simulink model "Sim_Multi"  (R2016b)
settings: Solver=ode3  StartTime=0.0  StopTime=sim_time  FixedStep=t_sim  MaxStep=t_control  RelTol=1e-5  EnableMultiTasking=on
values from neighbouring files (symbols this model uses):
  Att_init = [0;0;0] * d2r    [Init_Multi.m]
  Blade_flapping = 0    [Init_Multi.m]
  C_D = 0.40    (= 0.4)    [Init_Multi.m]
  CoG_nominal = [0;0;0.001]    [Init_Multi.m]
  CoG_real = [0;0;0.001]    [Init_Multi.m]
  Coriolis_correction = 1    [Init_Multi.m]
  d2r = pi/180    (= 0.0174532925199)    [Init_Multi.m]
  Dyn_thrust = 0    [Init_Multi.m]
  g = 9.80665    [Init_Multi.m]
  J_nominal = [Jxx Jxy Jxz;Jyx Jyy Jyz;Jzx Jzy Jzz]    [Init_Multi.m]
  J_real = [Jxx Jxy Jxz;Jyx Jyy Jyz;Jzx Jzy Jzz]    [Init_Multi.m]
  k1 = -1.125    [Init_Multi.m]
  k2 = -1.372    [Init_Multi.m]
  k3 = -1.718    [Init_Multi.m]
  k4 = -0.655    [Init_Multi.m]
  k_a1s = 1.5 / 4.0    (= 0.375)    [Init_Multi.m]
  k_beta = 0.23    [Init_Multi.m]
  kappa = 1.00    (= 1)    [Init_Multi.m]
  Kff_1 = 0.7*[1;1;0.95]    [Init_Multi.m]
  Ki_1 = 10*[1;1;1.5]    [Init_Multi.m]
  Kp_1 = 15*[1;1;1.5]    [Init_Multi.m]
  mass_nominal = 0.550    (= 0.55)    [Init_Multi.m]
  mass_real = 0.550    (= 0.55)    [Init_Multi.m]
  max_thrust = max_thrust + (MotorMatrix_nominal(i,7)*MotorMatrix_nominal(i,12)+MotorMatrix_nominal(i,8)*MotorMatrix_nominal(i,12)^2)    [Init_Multi.m]
  MaxRate_cmd = [360;360;120] * d2r    [Init_Multi.m]
  min_thrust = min_thrust + (MotorMatrix_nominal(i,7)*MotorMatrix_nominal(i,11)+MotorMatrix_nominal(i,8)*MotorMatrix_nominal(i,11)^2)    [Init_Multi.m]
  MotorMap = B' * inv(B * B')    [Init_Multi.m]
  MotorMatrix_nominal = [045 , 0.170 , -0.028 , -1 , 1.0 , 0.010 , [9.6820 , 0.010872]*1e-5 , [1.4504 , 0.0016312]*1e-6 , 0000 , 6000 , [0.0 , 0.0 , 0.0] , 8*2.54/100 , 11/1000;                         135 , 0.170 , -0.028 , +1 , 1.0 , 0.010 , [9.6820 , 0.010872]*1e-5 , [1.4504 , 0.0016312]*1e-6 , 0000 , 6000 , [0.0 , 0.0 , 0.0] , 8*2.54/100 , 11/1000;                         225 , 0.170 , -0.028 , -1 , 1.0 , 0.010 , [9. ...(+284 chars)    [Init_Multi.m]
  MotorMatrix_real = [045 , 0.170 , -0.028 , -1 , 1.0 , 0.010 , [9.6820 , 0.010872]*1e-5 , [1.4504 , 0.0016312]*1e-6 , 0000 , 6000 , [0.0 , 0.0 , 0.0] , 8*2.54/100 , 11/1000;                      135 , 0.170 , -0.028 , +1 , 1.0 , 0.010 , [9.6820 , 0.010872]*1e-5 , [1.4504 , 0.0016312]*1e-6 , 0000 , 6000 , [0.0 , 0.0 , 0.0] , 8*2.54/100 , 11/1000;                      225 , 0.170 , -0.028 , -1 , 1.0 , 0.010 , [9.6820 , ...(+275 chars)    [Init_Multi.m]
  Noise_flag = 0    [Init_Multi.m]
  omega_init = [0;0;0]    [Init_Multi.m]
  q_init = rpy2quat(Att_init)    [Init_Multi.m]
  r2d = 180/pi    (= 57.2957795131)    [Init_Multi.m]
  rho = 1.225    [Init_Multi.m]
  rpm2radpersec = 2*pi/60    (= 0.10471975512)    [Init_Multi.m]
  rpm_init = 3104.5025852    [Init_Multi.m]
  Surface_params = [a;b;c]    [Init_Multi.m]
  t_control = 1/500    (= 0.002)    [Init_Multi.m]
  t_sim = t_control/2    (= 0.001)    [Init_Multi.m]
  thrust_gain = (max_thrust - min_thrust) / 1000    (= 0)    [Init_Multi.m]
  thrust_offset = min_thrust    (= 0)    [Init_Multi.m]
  thrust_reserve = 0.10    (= 0.1)    [Init_Multi.m]
  v_h = 4.0    (= 4)    [Init_Multi.m]
  Vb_init = [0;0;0]    [Init_Multi.m]
  Vi_init = R_IB_init' * Vb_init    [Init_Multi.m]
  Xi_init = [0;0;0]    [Init_Multi.m]
undefined symbols (not defined in the file or in its folder): DiscIntNeverNeededParam, rpy2quat, thrust2rpm
libraries: simulink x17
(part 1 of 4)
settings Model: Creator=JV  LastModifiedBy=vervoorst
settings DataIOCC: LimitDataPoints=on  SaveFormat=Array  SignalLoggingSaveFormat=ModelDataLogs
settings OptimizationCC: ExpressionDepthLimit=2147483647  InitFltsAndDblsToZero=on  LifeSpan=inf
settings DebuggingCC: UnderspecifiedInitializationDetection=Classic  MergeDetectMultiDrivingBlocksExec=none  SolverPrmCheckMsg=warning  FcnCallInpInsideContextMsg=warning  StateNameClashWarn=warning  SFUnexpectedBacktrackingDiag=warning  SFNoUnconditionalDefaultTransitionDiag=warning  SFExecutionAtInitializationDiag=none
settings HardwareCC: ProdBitPerPointer=32  ProdBitPerSizeT=32  ProdBitPerPtrDiffT=32  ProdLargestAtomicFloat=None  ProdIntDivRoundTo=Undefined  ProdEndianess=Unspecified  ProdWordSize=32  ProdHWDeviceType=32-bit Generic
settings ModelReferenceCC: PropagateSignalLabelsOutOfModel=off
settings GRTTargetCC: TargetLangStandard=C89/C90 (ANSI)  GeneratePreprocessorConditionals=Disable all  CombineOutputUpdateFcns=off  GRTInterface=on
settings ConfigComp: CovMetricSettings=dw  CovHtmlReporting=on  CovSaveCumulativeToWorkspaceVar=on  CovSaveSingleToWorkspaceVar=on  CovExternalEMLEnable=off  CovSFcnEnable=off

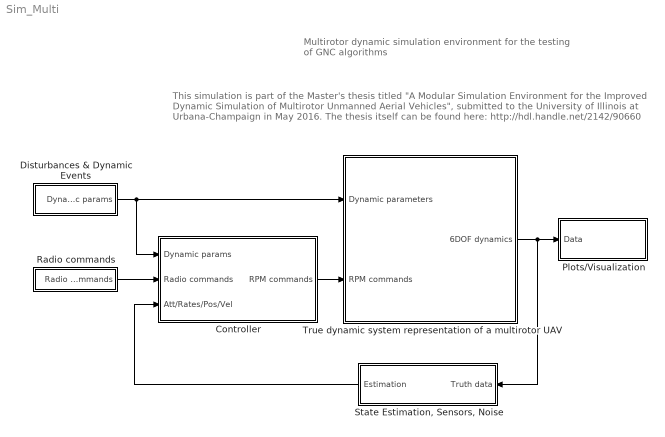
== system Sim_Multi ==
  note: This simulation is part of the Master's thesis titled "A Modular Simulation Environment for the Improved Dynamic Simulation
      | of Multirotor Unmanned Aerial Vehicles", submitted to the University of Illinois at Urbana-Champaign in May 2016.
      | The thesis itself can be found here: http://hdl.handle.net/2142/90660
  note: Multirotor dynamic simulation environment
      | for the testing of GNC algorithms
  Controller : Subsystem
  Disturbances & Dynamic Events : Subsystem
  Plots/Visualization : Subsystem
  Radio commands : Subsystem
  "State Estimation, Sensors, Noise" : Subsystem
  True dynamic system representation of a multirotor UAV : Subsystem
  wires:
  True dynamic system representation of a multirotor UAV/1(6DOF dynamics) -> Plots/Visualization/1(Data), "State Estimation, Sensors, Noise"/1(Truth data)
  Radio commands/1(Radio commands) -> Controller/2(Radio commands)
  "State Estimation, Sensors, Noise"/1(Estimation) -> Controller/3(Att/Rates/Pos/Vel)
  Controller/1(RPM commands) -> True dynamic system representation of a multirotor UAV/2(RPM commands)
  Disturbances & Dynamic Events/1(Dynamic params) -> True dynamic system representation of a multirotor UAV/1(Dynamic parameters), Controller/1(Dynamic params)

== system Sim_Multi/Controller ==
  note: All system parameters used in this block are the nominal parameters
      | that the controller is given about the system.
      | The true parameters of the dynamic system such as mass, inertia,
      | motor mapping matrix, ... may differ from these values.
  Dynamic params : Inport
  Radio commands : Inport  Port=2
  Att/Rates/Pos/Vel : Inport  Port=3
  Controller Structure : Subsystem
  Mapping thrust to rpm and saturation : Subsystem
  Motor mapping : Subsystem
  Reshape : Reshape  OutputDimensionality=Column vector (2-D)
  RPM commands : Outport
  tag scope: RPM_commands=global
  wires:
  Att/Rates/Pos/Vel/1 -> Controller Structure/2(Att/Rates/Pos/Vel)
  Controller Structure/1(Torques/thrust cmd) -> Motor mapping/1(Torques/thrust cmd)
  Radio commands/1 -> Controller Structure/1(Radio commands)
  Reshape/1 -> RPM commands/1
  Dynamic params/1 -> Controller Structure/3(Dynamic params), Mapping thrust to rpm and saturation/2(Dynamic parameters)
  Mapping thrust to rpm and saturation/1(RPM_cmd) -> [RPM_commands], Reshape/1
  Motor mapping/1(Thrust cmds) -> Mapping thrust to rpm and saturation/1(Thrust_cmds)

== system Sim_Multi/Disturbances & Dynamic Events ==
  Bus Creator : BusCreator  Inputs=12
  Constant : Constant  Value=MotorMatrix_real
  Constant1 : Constant  Value=CoG_real
  Constant2 : Constant  Value=mass_real
  Constant3 : Constant  Value=J_real
  Constant4 : Constant  Value=MotorMatrix_nominal
  Constant5 : Constant  Value=CoG_nominal
  Constant6 : Constant  Value=mass_nominal
  Constant7 : Constant  Value=J_nominal
  Disturbance (forces) : Constant  Value=0*[1;1;1]
  Disturbance (torques) : Constant  Value=0*[1;1;1]
  Surface area params : Constant  Value=Surface_params
  Wind vector : Constant  Value=[0;0;0]
  Dynamic params : Outport
  wires:
  Bus Creator/1 -> Dynamic params/1
  Constant/1 -> Bus Creator/1  "MotorMatrix_real"
  Constant1/1 -> Bus Creator/2  "CoG_real"
  Constant2/1 -> Bus Creator/3  "mass_real"
  Constant3/1 -> Bus Creator/4  "J_real"
  Surface area params/1 -> Bus Creator/12  "Surface_params"
  Disturbance (torques)/1 -> Bus Creator/11  "Moment_disturb"
  Disturbance (forces)/1 -> Bus Creator/10  "Force_disturb"
  Wind vector/1 -> Bus Creator/9  "Wind_i"
  Constant4/1 -> Bus Creator/5  "MotorMatrix_nominal"
  Constant5/1 -> Bus Creator/6  "CoG_nominal"
  Constant6/1 -> Bus Creator/7  "mass_nominal"
  Constant7/1 -> Bus Creator/8  "J_nominal"

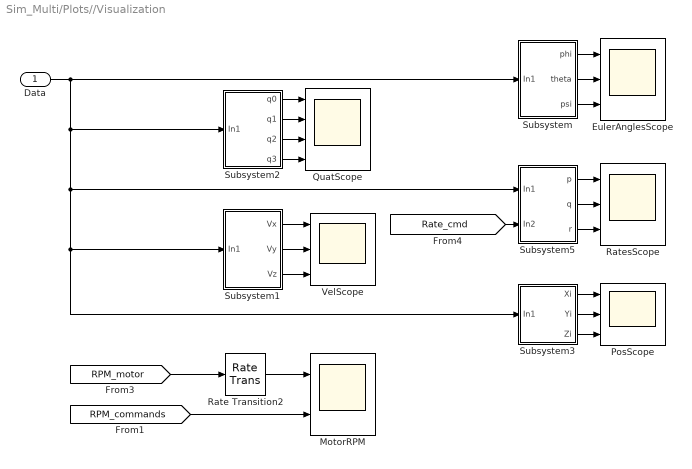
== system Sim_Multi/Plots//Visualization ==
  Data : Inport
  EulerAnglesScope : Scope  NumInputPorts=3
  MotorRPM : Scope  NumInputPorts=2
  PosScope : Scope  NumInputPorts=3
  QuatScope : Scope  NumInputPorts=4
  Rate Transition2 : RateTransition
  RatesScope : Scope  NumInputPorts=3
  Subsystem : Subsystem
  Subsystem1 : Subsystem
  Subsystem2 : Subsystem
  Subsystem3 : Subsystem
  Subsystem5 : Subsystem
  VelScope : Scope  NumInputPorts=3
  wires:
  Data/1 -> Subsystem3/1(In1), Subsystem1/1(In1), Subsystem5/1(In1), Subsystem2/1(In1), Subsystem/1(In1)
  Subsystem/1(phi) -> EulerAnglesScope/1
  Subsystem/2(theta) -> EulerAnglesScope/2
  Subsystem/3(psi) -> EulerAnglesScope/3
  Subsystem2/1(q0) -> QuatScope/1
  Subsystem2/2(q1) -> QuatScope/2
  Subsystem2/3(q2) -> QuatScope/3
  Subsystem2/4(q3) -> QuatScope/4
  Subsystem1/1(Vx) -> VelScope/1
  Subsystem1/2(Vy) -> VelScope/2
  Subsystem1/3(Vz) -> VelScope/3
  Subsystem3/2(Yi) -> PosScope/2
  Subsystem3/3(Zi) -> PosScope/3
  Subsystem3/1(Xi) -> PosScope/1
  Subsystem5/1(p) -> RatesScope/1
  Subsystem5/2(q) -> RatesScope/2
  Subsystem5/3(r) -> RatesScope/3
  [Rate_cmd] -> Subsystem5/2(In2)
  [RPM_commands] -> MotorRPM/2
  [RPM_motor] -> Rate Transition2/1
  Rate Transition2/1 -> MotorRPM/1

== system Sim_Multi/Radio commands ==
  Rate Transition : RateTransition  OutPortSampleTime=t_control
  Rate commands : Subsystem
  Radio commands : Outport
  wires:
  Rate commands/1(Rate commands) -> Rate Transition/1
  Rate Transition/1 -> Radio commands/1

== system Sim_Multi/State Estimation, Sensors, Noise ==
  Truth data : Inport
  Rate Transition : RateTransition  OutPortSampleTime=t_control
  Sensor models : Subsystem
  State estimation : Subsystem
  Estimation : Outport
  wires:
  State estimation/1(Att/Pos/Vel/Accel) -> Rate Transition/1
  Sensor models/1(Corrupted) -> State estimation/1(Sensors)
  Truth data/1 -> Sensor models/1(Truth)
  Rate Transition/1 -> Estimation/1

== system Sim_Multi/True dynamic system representation of a multirotor UAV ==
  Dynamic parameters : Inport
  RPM commands : Inport  Port=2
  6DOF model : Subsystem
  Bus Creator : BusCreator  Inputs=10
  Bus Selector : BusSelector  OutputSignals=mass_real,J_real
  Force/Moment computation : Subsystem
  Rate Transition : RateTransition  OutPortSampleTime=t_sim
  Rate Transition1 : RateTransition  X0=rpm_init  OutPortSampleTime=t_sim
  6DOF dynamics : Outport
  wires:
  RPM commands/1 -> Rate Transition1/1
  Bus Creator/1 -> Force/Moment computation/1(6DOF dynamics), 6DOF dynamics/1
  Dynamic parameters/1 -> Rate Transition/1
  6DOF model/1(X_i [m]) -> Bus Creator/1  "X_i"
  6DOF model/2(V_i [m/s]) -> Bus Creator/2  "V_i"
  6DOF model/3(V_b [m/s]) -> Bus Creator/3  "V_b"
  6DOF model/4(a_b [m/s^2]) -> Bus Creator/4  "a_b"
  Bus Selector/2 -> 6DOF model/4(Inertia [kgm^2])  "<J_real>"
  Bus Selector/1 -> 6DOF model/3(Mass [kg])  "<mass_real>"
  Force/Moment computation/1(Total forces) -> 6DOF model/1(Forces [N])
  Force/Moment computation/2(Total moments) -> 6DOF model/2(Moments [Nm])
  Rate Transition1/1 -> Force/Moment computation/2(RPM commands)
  Rate Transition/1 -> Bus Selector/1, Force/Moment computation/3(Dynamic parameters)
  6DOF model/5(a_i [m/s^2]) -> Bus Creator/5  "a_i"
  6DOF model/6(DCM_ib) -> Bus Creator/6  "DCM_ib"
  6DOF model/7(Quaternion q) -> Bus Creator/7  "Quat q"
  6DOF model/8(Euler [rad]) -> Bus Creator/8  "Euler"
  6DOF model/9(omega [rad/s]) -> Bus Creator/9  "omega"
  6DOF model/10(omega_dot [rad/s^2]) -> Bus Creator/10  "omega_dot"

== system Sim_Multi/Controller/Controller Structure ==
  Radio commands : Inport
  Att/Rates/Pos/Vel : Inport  Port=2
  Dynamic params : Inport  Port=3
  Bus Selector : BusSelector  OutputSignals=J_nominal
  Inner-loop control only : Subsystem
  Torques/thrust cmd : Outport
  tag scope: J_control=global
  wires:
  Dynamic params/1 -> Bus Selector/1
  Bus Selector/1 -> [J_control]  "<J_nominal>"
  Radio commands/1 -> Inner-loop control only/2(Radio commands)
  Att/Rates/Pos/Vel/1 -> Inner-loop control only/1(Att/Rates/Pos/Vel)
  Inner-loop control only/1(Control out) -> Torques/thrust cmd/1

== system Sim_Multi/Controller/Mapping thrust to rpm and saturation ==
  Thrust_cmds : Inport
  Dynamic parameters : Inport  Port=2
  Bus Selector1 : BusSelector  OutputSignals=MotorMatrix_nominal
  For Each Subsystem : Subsystem  TreatAsAtomicUnit=on
  Rate Transition : RateTransition  OutPortSampleTime=t_control
  RPM_cmd : Outport
  wires:
  For Each Subsystem/1(RPM_cmd_sat) -> Rate Transition/1
  Dynamic parameters/1 -> Bus Selector1/1
  Bus Selector1/1 -> For Each Subsystem/2(MotorMatrix_nominal)  "<MotorMatrix_nominal>"
  Rate Transition/1 -> RPM_cmd/1
  Thrust_cmds/1 -> For Each Subsystem/1(Thrust_cmds)

== system Sim_Multi/Controller/Motor mapping ==
  note: Overall thrust command is limited to a range
      | of 10...90% of max thrust to still allow room
      | for torque demands needed for maneuvering
  note: The motor mapping matrix used here to transform body axis torque commands
      | into thrust commands for each motor is populated with the nominal arm length
      | and motor position information that the controller thinks are correct, not the
      | actual values used in the true dynamics computation block.
  Torques/thrust cmd : Inport
  Constant1 : Constant  Value=MotorMap
  Demux : Demux  Outputs=[3 1]
  Matrix Multiply1 : Product  Multiplication=Matrix(*)
  Max thrust limit : Subsystem
  Min thrust limit : Subsystem
  Mux : Mux  Inputs=2
  Rate Transition : RateTransition  OutPortSampleTime=t_control
  Saturation Dynamic : simulink/Discontinuities/Saturation Dynamic  OutMin=[]  OutMax=[]  OutDataTypeStr=Inherit: Same as second input  OutDataType=fixdt(1, 16)  OutScaling=2^-10  DoSatur=off
  Thrust cmds : Outport
  wires:
  Constant1/1 -> Matrix Multiply1/1
  Rate Transition/1 -> Thrust cmds/1  "These are thrust demands to each motor"
  Matrix Multiply1/1 -> Rate Transition/1
  Torques/thrust cmd/1 -> Demux/1
  Demux/2 -> Saturation Dynamic/2
  Min thrust limit/1(Out1) -> Saturation Dynamic/3
  Max thrust limit/1(Out1) -> Saturation Dynamic/1
  Saturation Dynamic/1 -> Mux/2
  Demux/1 -> Mux/1
  Mux/1 -> Matrix Multiply1/2

== system Sim_Multi/Plots//Visualization/Subsystem ==
  In1 : Inport
  Bus Selector : BusSelector  OutputSignals=Euler
  Demux : Demux  Outputs=3
  Gain : Gain  Gain=r2d
  phi : Outport
  theta : Outport  Port=2
  psi : Outport  Port=3
  wires:
  Bus Selector/1 -> Gain/1  "<Euler>"
  In1/1 -> Bus Selector/1
  Gain/1 -> Demux/1
  Demux/1 -> phi/1
  Demux/2 -> theta/1
  Demux/3 -> psi/1

== system Sim_Multi/Plots//Visualization/Subsystem1 ==
  In1 : Inport
  Bus Selector : BusSelector  OutputSignals=V_i
  Demux4 : Demux  Outputs=3
  Vx : Outport
  Vy : Outport  Port=2
  Vz : Outport  Port=3
  wires:
  Bus Selector/1 -> Demux4/1  "<V_i>"
  In1/1 -> Bus Selector/1
  Demux4/1 -> Vx/1
  Demux4/2 -> Vy/1
  Demux4/3 -> Vz/1

== system Sim_Multi/Plots//Visualization/Subsystem2 ==
  In1 : Inport
  Bus Selector : BusSelector  OutputSignals=Quat q
  Demux5 : Demux
  q0 : Outport
  q1 : Outport  Port=2
  q2 : Outport  Port=3
  q3 : Outport  Port=4
  wires:
  Bus Selector/1 -> Demux5/1  "<Quat q>"
  In1/1 -> Bus Selector/1
  Demux5/1 -> q0/1
  Demux5/2 -> q1/1
  Demux5/3 -> q2/1
  Demux5/4 -> q3/1

== system Sim_Multi/Plots//Visualization/Subsystem3 ==
  In1 : Inport
  Bus Selector : BusSelector  OutputSignals=X_i
  Demux4 : Demux  Outputs=3
  Xi : Outport
  Yi : Outport  Port=2
  Zi : Outport  Port=3
  wires:
  Bus Selector/1 -> Demux4/1  "<X_i>"
  In1/1 -> Bus Selector/1
  Demux4/1 -> Xi/1
  Demux4/2 -> Yi/1
  Demux4/3 -> Zi/1

== system Sim_Multi/Plots//Visualization/Subsystem5 ==
  In1 : Inport
  In2 : Inport  Port=2
  Bus Selector : BusSelector  OutputSignals=omega
  Demux : Demux  Outputs=3
  Demux1 : Demux  Outputs=3
  Mux : Mux  Inputs=2
  Mux1 : Mux  Inputs=2
  Mux2 : Mux  Inputs=2
  Rate Transition : RateTransition  OutPortSampleTime=t_sim
  p : Outport
  q : Outport  Port=2
  r : Outport  Port=3
  wires:
  Bus Selector/1 -> Demux/1  "<omega>"
  Demux/1 -> Mux1/1
  Demux1/1 -> Mux1/2
  Demux/2 -> Mux/1
  Demux1/2 -> Mux/2
  Demux/3 -> Mux2/1
  Demux1/3 -> Mux2/2
  In1/1 -> Bus Selector/1
  In2/1 -> Rate Transition/1
  Mux1/1 -> p/1
  Mux/1 -> q/1
  Mux2/1 -> r/1
  Rate Transition/1 -> Demux1/1

== system Sim_Multi/Radio commands/Rate commands ==
  note: The signal magnitude for the throttle should be
      | in a range of [0,1000]
  Filter : Subsystem
  Mux : Mux  Inputs=3
  Mux1 : Mux  Inputs=2
  Pitch rate signal : Subsystem
  Rate Transition : RateTransition  OutPortSampleTime=t_control
  Roll rate signal : Subsystem
  Throttle value : Constant  Value=299.9916292904752
  Yaw rate signal : Subsystem
  Rate commands : Outport
  wires:
  Filter/2(theta_dot filtered) -> Mux/2
  Mux1/1 -> Rate commands/1
  Filter/3(psi_dot filtered) -> Mux/3
  Filter/1(phi_dot filtered) -> Mux/1
  Roll rate signal/1(phi) -> Filter/1(Roll rate)
  Mux/1 -> Rate Transition/1
  Pitch rate signal/1(theta) -> Filter/2(Pitch rate)
  Yaw rate signal/1(psi) -> Filter/3(Yaw rate)
  Throttle value/1 -> Mux1/2
  Rate Transition/1 -> Mux1/1

== system Sim_Multi/State Estimation, Sensors, Noise/Sensor models ==
  note: The available sensor outputs are body rates and body accelerations.
      | In the simple case, noise is added to the rate and accel outputs of the 6DOF block to 'simulate' sensor output.
  Truth : Inport
  Acc noise : Subsystem
  Bus Creator : BusCreator  Inputs=9
  Bus Selector : BusSelector  OutputSignals=a_b,omega
  Bus Selector1 : BusSelector  OutputSignals=X_i,V_i,V_b,DCM_ib,Quat q,Euler,omega_dot
  Gain : Gain
  Gain1 : Gain
  Gyro noise : Subsystem
  Noisy acc : Scope
  Noisy omega : Scope
  Sum : Sum
  Sum1 : Sum
  Corrupted : Outport
  wires:
  Truth/1 -> Bus Selector/1, Bus Selector1/1
  Bus Creator/1 -> Corrupted/1
  Sum/1 -> Noisy omega/1, Gain/1  "omega"
  Sum1/1 -> Noisy acc/1, Gain1/1  "a_b"
  Bus Selector1/1 -> Bus Creator/1  "<X_i>"
  Bus Selector1/2 -> Bus Creator/2  "<V_i>"
  Bus Selector1/3 -> Bus Creator/3  "<V_b>"
  Acc noise/1(Noise) -> Sum1/1
  Bus Selector/1 -> Sum1/2  "<a_b>"
  Gain1/1 -> Bus Creator/4  "a_b"
  Bus Selector1/4 -> Bus Creator/5  "<DCM_ib>"
  Bus Selector1/5 -> Bus Creator/6  "<Quat q>"
  Bus Selector1/6 -> Bus Creator/7  "<Euler>"
  Gyro noise/1(Noise) -> Sum/2
  Bus Selector/2 -> Sum/1  "<omega>"
  Gain/1 -> Bus Creator/8  "omega"
  Bus Selector1/7 -> Bus Creator/9  "<omega_dot>"

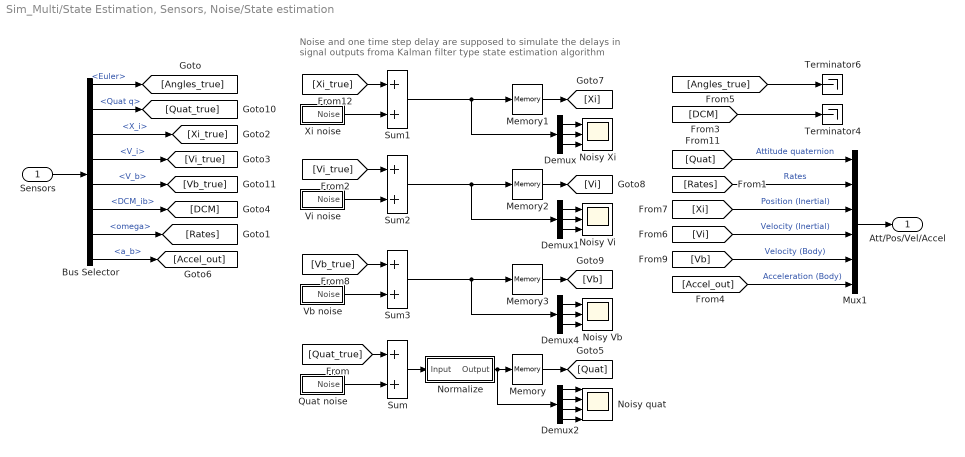
== system Sim_Multi/State Estimation, Sensors, Noise/State estimation ==
  note: Noise and one time step delay are supposed to simulate the delays
      | in signal outputs froma Kalman filter type state estimation algorithm
  Sensors : Inport
  Bus Selector : BusSelector  OutputSignals=Euler,Quat q,X_i,V_i,V_b,DCM_ib,omega,a_b
  Demux : Demux  Outputs=3
  Demux1 : Demux  Outputs=3
  Demux2 : Demux
  Demux4 : Demux  Outputs=3
  Memory : Memory  X0=q_init
  Memory1 : Memory  X0=Xi_init
  Memory2 : Memory  X0=Vi_init
  Memory3 : Memory  X0=Vi_init
  Mux1 : Mux  Inputs=6
  Noisy Vb : Scope  NumInputPorts=3
  Noisy Vi : Scope  NumInputPorts=3
  Noisy Xi : Scope  NumInputPorts=3
  Noisy quat : Scope  NumInputPorts=4
  Normalize : Subsystem
  Quat noise : Subsystem
  Sum{,1..3} (4 alike) : Sum
  Terminator4 : Terminator
  Terminator6 : Terminator
  Vb noise : Subsystem
  Vi noise : Subsystem
  Xi noise : Subsystem
  Att/Pos/Vel/Accel : Outport
  wires:
  Sensors/1 -> Bus Selector/1
  Bus Selector/3 -> [Xi_true]  "<X_i>"
  Bus Selector/4 -> [Vi_true]  "<V_i>"
  Bus Selector/6 -> [DCM]  "<DCM_ib>"
  Bus Selector/7 -> [Rates]  "<omega>"
  Bus Selector/8 -> [Accel_out]  "<a_b>"
  Bus Selector/1 -> [Angles_true]  "<Euler>"
  [Quat] -> Mux1/1  "Attitude quaternion"
  [Rates] -> Mux1/2  "Rates"
  Bus Selector/2 -> [Quat_true]  "<Quat q>"
  [DCM] -> Terminator4/1
  [Angles_true] -> Terminator6/1
  Sum/1 -> Normalize/1(Input)
  Quat noise/1(Noise) -> Sum/2
  [Quat_true] -> Sum/1
  Normalize/1(Output) -> Demux2/1, Memory/1
  Memory/1 -> [Quat]
  Xi noise/1(Noise) -> Sum1/2
  Sum1/1 -> Demux/1, Memory1/1
  Memory1/1 -> [Xi]
  [Xi_true] -> Sum1/1
  Vi noise/1(Noise) -> Sum2/2
  Memory2/1 -> [Vi]
  [Vi_true] -> Sum2/1
  [Xi] -> Mux1/3  "Position (Inertial)"
  [Vi] -> Mux1/4  "Velocity (Inertial)"
  Mux1/1 -> Att/Pos/Vel/Accel/1
  Sum2/1 -> Demux1/1, Memory2/1
  Demux/1 -> Noisy Xi/1
  Demux/2 -> Noisy Xi/2
  Demux/3 -> Noisy Xi/3
  Demux1/1 -> Noisy Vi/1
  Demux1/2 -> Noisy Vi/2
  Demux1/3 -> Noisy Vi/3
  Demux2/1 -> Noisy quat/1
  Demux2/2 -> Noisy quat/2
  Demux2/3 -> Noisy quat/3
  Demux2/4 -> Noisy quat/4
  Vb noise/1(Noise) -> Sum3/2
  Memory3/1 -> [Vb]
  [Vb_true] -> Sum3/1
  Sum3/1 -> Demux4/1, Memory3/1
  Demux4/1 -> Noisy Vb/1
  Demux4/2 -> Noisy Vb/2
  Demux4/3 -> Noisy Vb/3
  Bus Selector/5 -> [Vb_true]  "<V_b>"
  [Vb] -> Mux1/5  "Velocity (Body)"
  [Accel_out] -> Mux1/6  "Acceleration (Body)"

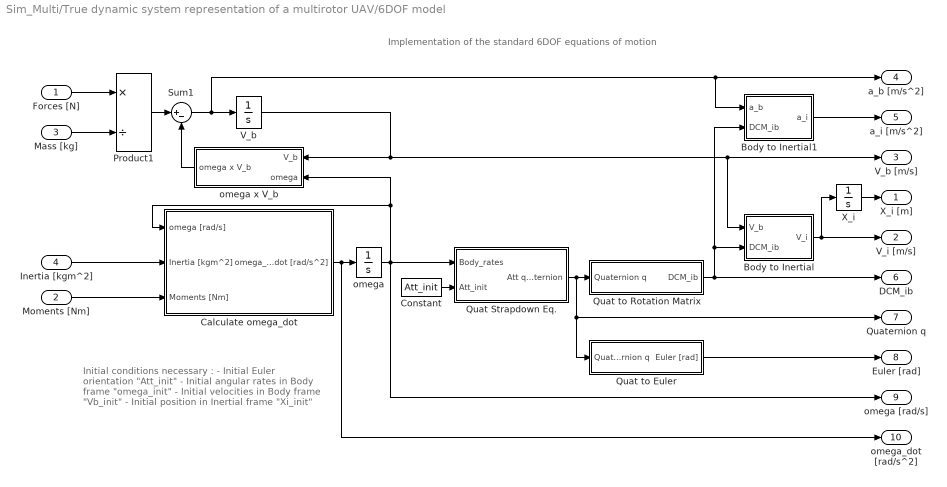
== system Sim_Multi/True dynamic system representation of a multirotor UAV/6DOF model ==
  note: Implementation of the standard 6DOF equations of motion
  note: Initial conditions necessary :
      | - Initial Euler orientation "Att_init"
      | - Initial angular rates in Body frame "omega_init"
      | - Initial velocities in Body frame "Vb_init"
      | - Initial position in Inertial frame "Xi_init"
  Forces [N] : Inport
  Moments [Nm] : Inport  Port=2
  Mass [kg] : Inport  Port=3
  Inertia [kgm^2] : Inport  Port=4
  Body to Inertial : Subsystem
  Body to Inertial1 : Subsystem
  Calculate omega_dot : Subsystem
  Constant : Constant  Value=Att_init
  Product1 : Product  Inputs=*/  SaturateOnIntegerOverflow=on  OutDataTypeStr=Inherit: Same as first input
  Quat Strapdown Eq. : Subsystem
  Quat to Euler : Subsystem
  Quat to Rotation Matrix : Subsystem
  Sum1 : Sum  Inputs=|+-  SaturateOnIntegerOverflow=on
  V_b : Integrator  InitialCondition=Vb_init
  X_i : Integrator  InitialCondition=Xi_init
  omega : Integrator  InitialCondition=omega_init
  omega x V_b : Subsystem
  X_i [m] : Outport
  V_i [m/s] : Outport  Port=2
  V_b [m/s] : Outport  Port=3
  a_b [m/s^2] : Outport  Port=4
  a_i [m/s^2] : Outport  Port=5
  DCM_ib : Outport  Port=6
  Quaternion q : Outport  Port=7
  Euler [rad] : Outport  Port=8
  omega [rad/s] : Outport  Port=9
  omega_dot [rad/s^2] : Outport  Port=10
  wires:
  Forces [N]/1 -> Product1/1
  Mass [kg]/1 -> Product1/2
  Product1/1 -> Sum1/1
  omega x V_b/1(omega x V_b) -> Sum1/2
  V_b/1 -> V_b [m/s]/1, Body to Inertial/1(V_b), omega x V_b/1(V_b)
  Inertia [kgm^2]/1 -> Calculate omega_dot/2(Inertia [kgm^2])
  Moments [Nm]/1 -> Calculate omega_dot/3(Moments [Nm])
  Calculate omega_dot/1(omega_dot [rad/s^2]) -> omega_dot [rad/s^2]/1, omega/1
  omega/1 -> Calculate omega_dot/1(omega [rad/s]), omega x V_b/2(omega), omega [rad/s]/1, Quat Strapdown Eq./1(Body_rates)
  Quat Strapdown Eq./1(Att quaternion) -> Quat to Euler/1(Quaternion q), Quaternion q/1, Quat to Rotation Matrix/1(Quaternion q)
  Quat to Euler/1(Euler [rad]) -> Euler [rad]/1
  Body to Inertial/1(V_i) -> V_i [m/s]/1, X_i/1
  X_i/1 -> X_i [m]/1
  Constant/1 -> Quat Strapdown Eq./2(Att_init)
  Quat to Rotation Matrix/1(DCM_ib) -> Body to Inertial1/2(DCM_ib), Body to Inertial/2(DCM_ib), DCM_ib/1
  Body to Inertial1/1(a_i) -> a_i [m/s^2]/1
  Sum1/1 -> V_b/1, a_b [m/s^2]/1, Body to Inertial1/1(a_b)

== system Sim_Multi/True dynamic system representation of a multirotor UAV/Force//Moment computation ==
  note: Computation of all forces and moments acting on the airframe
  6DOF dynamics : Inport
  RPM commands : Inport  Port=2
  Dynamic parameters : Inport  Port=3
  Bus Selector : BusSelector  OutputSignals=Force_disturb,Moment_disturb
  Compute aerodynamic drag of the airframe in Body axes : Subsystem
  Compute force of gravity in Body axes : Subsystem
  Forces and moments generated by spinning propellers : Subsystem
  Sum{,1..3} (4 alike) : Sum  Inputs=|++
  Total forces : Outport
  Total moments : Outport  Port=2
  wires:
  RPM commands/1 -> Forces and moments generated by spinning propellers/1(RPM_commands)
  6DOF dynamics/1 -> Forces and moments generated by spinning propellers/3(6DOF dynamics), Compute aerodynamic drag of the airframe in Body axes/1(6DOF dynamics), Compute force of gravity in Body axes/1(6DOF dynamics)
  Forces and moments generated by spinning propellers/2(Motor forces) -> Sum/1
  Compute force of gravity in Body axes/1(Gravity force) -> Sum/2
  Dynamic parameters/1 -> Bus Selector/1, Compute aerodynamic drag of the airframe in Body axes/2(Dynamic parameters), Compute force of gravity in Body axes/2(Dynamic parameters), Forces and moments generated by spinning propellers/2(Dynamic parameters)
  Bus Selector/1 -> Sum1/2  "<Force_disturb>"
  Bus Selector/2 -> Sum2/2  "<Moment_disturb>"
  Forces and moments generated by spinning propellers/1(Motor moments) -> Sum2/1
  Sum/1 -> Sum3/1
  Sum3/1 -> Sum1/1
  Compute aerodynamic drag of the airframe in Body axes/1(Drag force) -> Sum3/2
  Sum2/1 -> Total moments/1
  Sum1/1 -> Total forces/1

== system Sim_Multi/Controller/Controller Structure/Inner-loop control only ==
  note: The output of the inner-loop controller is always
      | a set of three commanded torques around the
      | Body axes, roll/pitch/yaw, and an overall thrust
      | command.
      | This is independent of what the structure of the
      | multirotor airframe is assumed to be.
  Att/Rates/Pos/Vel : Inport
  Radio commands : Inport  Port=2
  Conversion stick values to rate commands : Subsystem
  Demux : Demux  Outputs=[4 3 3 3 3 3]
  PI Rate controller : Subsystem
  Terminator{,1..4} (5 alike) : Terminator
  Control out : Outport
  wires:
  Att/Rates/Pos/Vel/1 -> Demux/1
  Demux/3 -> Terminator/1  "Xi"
  Demux/4 -> Terminator1/1  "Vi"
  Demux/5 -> Terminator2/1  "Vb"
  Demux/6 -> Terminator3/1  "a_b"
  Radio commands/1 -> Conversion stick values to rate commands/1(Sticks/Throttle cmd)
  PI Rate controller/1(Control/Throttle out) -> Control out/1
  Demux/2 -> PI Rate controller/2(Rate_est)
  Conversion stick values to rate commands/1(Rates/Throttle cmd) -> PI Rate controller/1(Rates/Throttle cmd)
  Demux/1 -> Terminator4/1

== system Sim_Multi/Controller/Mapping thrust to rpm and saturation/For Each Subsystem ==
  note: The thrust commands from the controller are turned into RPM commands by solving the
      | nominal (quadratic) rpm to thrust equations for RPM.
      | These min and max RPM values are then saturated using the nominal min and max RPM
      | values given for the particular motor/propeller combination.
  Thrust_cmds : Inport  Partition=on  PartitionDimension=1  PartitionWidth=1
  MotorMatrix_nominal : Inport  Port=2  Partition=on  PartitionDimension=1  PartitionWidth=1
  For Each : ForEach  DisableCoverage=on  IndexMode=One-based
  Mux : Mux  Inputs=2
  Saturation Dynamic : simulink/Discontinuities/Saturation Dynamic  OutMin=[]  OutMax=[]  OutDataTypeStr=Inherit: Same as second input  OutDataType=fixdt(1, 16)  OutScaling=2^-10  DoSatur=off
  Saturation limit: no negative thrust : Saturate  UpperLimit=inf  LowerLimit=0
  Selector1 : Selector  InputPortWidth=17  IndexOptions=Index vector (dialog)  Indices=[11]  OutputSizes=1
  Selector2 : Selector  InputPortWidth=17  IndexOptions=Index vector (dialog)  Indices=[12]  OutputSizes=1
  Selector3 : Selector  InputPortWidth=17  IndexOptions=Index vector (dialog)  Indices=[7 8]  OutputSizes=1
  thrust2rpm : MATLABFcn  MATLABFcn=thrust2rpm(u)  OutputDimensions=1
  RPM_cmd_sat : Outport  ConcatenationDimension=1
  wires:
  Selector3/1 -> Mux/1  "Thrust params a1 and a2"
  Thrust_cmds/1 -> Saturation limit: no negative thrust/1
  Mux/1 -> thrust2rpm/1
  thrust2rpm/1 -> Saturation Dynamic/2  "Commanded RPM value for each motor"
  Selector2/1 -> Saturation Dynamic/1  "Nominal max RPM"
  Selector1/1 -> Saturation Dynamic/3  "Nominal min RPM"
  Saturation Dynamic/1 -> RPM_cmd_sat/1
  MotorMatrix_nominal/1 -> Selector1/1, Selector2/1, Selector3/1
  Saturation limit: no negative thrust/1 -> Mux/2

== system Sim_Multi/Controller/Motor mapping/Max thrust limit ==
  Constant : Constant  Value=max_thrust
  Constant2 : Constant  Value=min_thrust
  Gain : Gain  Gain=thrust_reserve
  Sum : Sum  Inputs=|+-
  Sum1 : Sum  Inputs=+-|
  Out1 : Outport
  wires:
  Constant/1 -> Sum1/1, Sum/1
  Sum1/1 -> Out1/1
  Constant2/1 -> Sum/2
  Sum/1 -> Gain/1
  Gain/1 -> Sum1/2

== system Sim_Multi/Controller/Motor mapping/Min thrust limit ==
  Constant : Constant  Value=max_thrust
  Constant2 : Constant  Value=min_thrust
  Gain : Gain  Gain=thrust_reserve
  Sum : Sum  Inputs=|+-
  Sum1 : Sum  Inputs=|++
  Out1 : Outport
  wires:
  Constant/1 -> Sum/1
  Sum1/1 -> Out1/1
  Constant2/1 -> Sum1/2, Sum/2
  Sum/1 -> Gain/1
  Gain/1 -> Sum1/1

== system Sim_Multi/Radio commands/Rate commands/Filter ==
  Roll rate : Inport
  Pitch rate : Inport  Port=2
  Yaw rate : Inport  Port=3
  Transfer Fcn{1..6} (6 alike) : TransferFcn  Denominator=[.01 1]
  phi_dot filtered : Outport
  theta_dot filtered : Outport  Port=2
  psi_dot filtered : Outport  Port=3
  wires:
  Transfer Fcn6/1 -> Transfer Fcn1/1
  Transfer Fcn2/1 -> Transfer Fcn3/1
  Transfer Fcn4/1 -> Transfer Fcn5/1
  Yaw rate/1 -> Transfer Fcn2/1
  Transfer Fcn3/1 -> psi_dot filtered/1
  Pitch rate/1 -> Transfer Fcn4/1
  Transfer Fcn5/1 -> theta_dot filtered/1
  Roll rate/1 -> Transfer Fcn6/1
  Transfer Fcn1/1 -> phi_dot filtered/1

== system Sim_Multi/Radio commands/Rate commands/Pitch rate signal ==
  note: The signal magnitude for the pitch channel should be at most 1.
      | It then gets scaled by a factor of 500 to simulate a PWM output
      | range of [-500,500]
  Add1 : Sum  Inputs=+++
  Add2 : Sum  Inputs=+++
  Constant : Constant  Value=0
  Gain : Gain
  Gain1 : Gain  Gain=0.1
  Gain2 : Gain  Gain=500
  Manual Switch : ManualSwitch  CurrentSetting=0
  Manual Switch1 : ManualSwitch
  Step1 : Step  SampleTime=0
  Step2 : Step  Time=2  After=-2  SampleTime=0
  Step3 : Step  Time=3.5  SampleTime=0
  Step4 : Step  Time=4.5  After=-2  SampleTime=0
  Step5 : Step  Time=5.5  SampleTime=0
  Step6 : Step  Time=3  SampleTime=0
  theta : Outport
  wires:
  Add1/1 -> Gain/1
  Step3/1 -> Add1/1
  Step4/1 -> Add1/2
  Step5/1 -> Add1/3
  Gain2/1 -> theta/1
  Gain/1 -> Manual Switch/1
  Add2/1 -> Gain1/1
  Step1/1 -> Add2/1
  Step2/1 -> Add2/2
  Step6/1 -> Add2/3
  Gain1/1 -> Manual Switch/2
  Manual Switch/1 -> Manual Switch1/1
  Constant/1 -> Manual Switch1/2
  Manual Switch1/1 -> Gain2/1

== system Sim_Multi/Radio commands/Rate commands/Roll rate signal ==
  note: The signal magnitude for the roll channel should be at most 1.
      | It then gets scaled by a factor of 500 to simulate a PWM output
      | range of [-500,500]
  Add : Sum  Inputs=+++
  Constant : Constant  Value=0
  Gain : Gain  Gain=0.1
  Gain2 : Gain  Gain=500
  Manual Switch : ManualSwitch
  Manual Switch1 : ManualSwitch
  Step : Step  Time=0.5  SampleTime=0
  Step1 : Step  Time=1.5  After=-2  SampleTime=0
  Step2 : Step  Time=2.5  SampleTime=0
  Step3 : Step  Time=0.5  SampleTime=0
  phi : Outport
  wires:
  Step/1 -> Add/1
  Step1/1 -> Add/2
  Step2/1 -> Add/3
  Add/1 -> Gain/1
  Gain2/1 -> phi/1
  Gain/1 -> Manual Switch/1
  Manual Switch/1 -> Manual Switch1/1
  Manual Switch1/1 -> Gain2/1
  Constant/1 -> Manual Switch1/2
  Step3/1 -> Manual Switch/2

== system Sim_Multi/Radio commands/Rate commands/Yaw rate signal ==
  note: The signal magnitude for the yaw channel should be at most 1.
      | It then gets scaled by a factor of 500 to simulate a PWM output
      | range of [-500,500]
  Add1 : Sum  Inputs=+++
  Add2 : Sum  Inputs=+++
  Constant : Constant  Value=0
  Gain : Gain  Gain=0.2
  Gain1 : Gain  Gain=0.2
  Gain2 : Gain  Gain=500
  Manual Switch : ManualSwitch  CurrentSetting=0
  Manual Switch1 : ManualSwitch  CurrentSetting=0
  Step1 : Step  Time=2  SampleTime=0
  Step2 : Step  Time=3  After=-2  SampleTime=0
  Step3 : Step  Time=4  SampleTime=0
  Step6 : Step  Time=6.5  SampleTime=0
  Step7 : Step  Time=7.5  After=-2  SampleTime=0
  Step8 : Step  Time=8.5  SampleTime=0
  psi : Outport
  wires:
  Step6/1 -> Add2/1
  Step7/1 -> Add2/2
  Step8/1 -> Add2/3
  Add2/1 -> Gain1/1
  Gain2/1 -> psi/1
  Step1/1 -> Add1/1
  Step2/1 -> Add1/2
  Step3/1 -> Add1/3
  Add1/1 -> Gain/1
  Gain/1 -> Manual Switch/2
  Manual Switch/1 -> Manual Switch1/1
  Manual Switch1/1 -> Gain2/1
  Constant/1 -> Manual Switch1/2
  Gain1/1 -> Manual Switch/1

== system Sim_Multi/State Estimation, Sensors, Noise/Sensor models/Acc noise ==
  Band-Limited White Noise : simulink/Sources/Band-Limited White Noise  Cov=t_sim*57.3*57.3/10000  Ts=t_sim  seed=[25341]
  Constant : Constant  Value=Noise_flag
  Constant1 : Constant  Value=0
  Gain1 : Gain  Gain=0.1
  Gain2 : Gain  Gain=0.08
  Integrator : Integrator
  Sum1 : Sum  Inputs=++|
  Switch : Switch  Criteria=u2 > Threshold
  Uniform Random Number : UniformRandomNumber  Minimum=-.001  Maximum=.001  Seed=657  SampleTime=t_sim
  Noise : Outport
  wires:
  Band-Limited White Noise/1 -> Gain2/1
  Uniform Random Number/1 -> Integrator/1
  Integrator/1 -> Gain1/1
  Switch/1 -> Noise/1
  Constant/1 -> Switch/2
  Constant1/1 -> Switch/3
  Gain2/1 -> Sum1/1
  Gain1/1 -> Sum1/2
  Sum1/1 -> Switch/1

== system Sim_Multi/State Estimation, Sensors, Noise/Sensor models/Gyro noise ==
  Band-Limited White Noise : simulink/Sources/Band-Limited White Noise  Cov=t_sim*57.3*57.3/10000  Ts=t_sim  seed=[23341]
  Constant : Constant  Value=Noise_flag
  Constant1 : Constant  Value=0
  Gain1 : Gain  Gain=0.1
  Gain2 : Gain  Gain=0.07
  Integrator : Integrator
  Sum1 : Sum  Inputs=++|
  Switch : Switch  Criteria=u2 > Threshold
  Uniform Random Number : UniformRandomNumber  Minimum=-.001  Maximum=.001  Seed=338  SampleTime=t_sim
  Noise : Outport
  wires:
  Band-Limited White Noise/1 -> Gain2/1
  Uniform Random Number/1 -> Integrator/1
  Integrator/1 -> Gain1/1
  Switch/1 -> Noise/1
  Constant/1 -> Switch/2
  Constant1/1 -> Switch/3
  Gain2/1 -> Sum1/1
  Gain1/1 -> Sum1/2
  Sum1/1 -> Switch/1

== system Sim_Multi/State Estimation, Sensors, Noise/State estimation/Normalize ==
  Input : Inport
  Divide : Product  Inputs=*/
  norm : Subsystem
  Output : Outport
  wires:
  Input/1 -> Divide/1, norm/1(u)
  norm/1(||u||) -> Divide/2
  Divide/1 -> Output/1

== system Sim_Multi/State Estimation, Sensors, Noise/State estimation/Quat noise ==
  Band-Limited White Noise : simulink/Sources/Band-Limited White Noise  Cov=t_sim*57.3*57.3/10000  Ts=t_sim*30  seed=[23099]
  Constant : Constant  Value=Noise_flag
  Constant1 : Constant  Value=0
  Gain2 : Gain  Gain=0.1
  Rate Transition1 : RateTransition  OutPortSampleTime=t_sim
  Switch : Switch  Criteria=u2 > Threshold
  Noise : Outport
  wires:
  Band-Limited White Noise/1 -> Gain2/1
  Switch/1 -> Noise/1
  Constant/1 -> Switch/2
  Constant1/1 -> Switch/3
  Gain2/1 -> Rate Transition1/1
  Rate Transition1/1 -> Switch/1

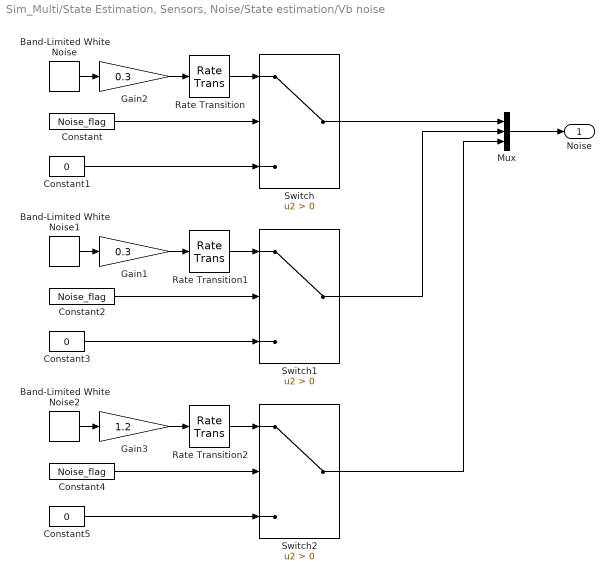
== system Sim_Multi/State Estimation, Sensors, Noise/State estimation/Vb noise ==
  Band-Limited White Noise : simulink/Sources/Band-Limited White Noise  Cov=t_sim*57.3*57.3/10000  Ts=t_sim*10  seed=[21234]
  Band-Limited White Noise1 : simulink/Sources/Band-Limited White Noise  Cov=t_sim*57.3*57.3/10000  Ts=t_sim*10  seed=[21234]
  Band-Limited White Noise2 : simulink/Sources/Band-Limited White Noise  Cov=t_sim*57.3*57.3/10000  Ts=t_sim*10  seed=[21234]
  Constant : Constant  Value=Noise_flag
  Constant1 : Constant  Value=0
  Constant2 : Constant  Value=Noise_flag
  Constant3 : Constant  Value=0
  Constant4 : Constant  Value=Noise_flag
  Constant5 : Constant  Value=0
  Gain1 : Gain  Gain=0.3
  Gain2 : Gain  Gain=0.3
  Gain3 : Gain  Gain=1.2
  Mux : Mux  Inputs=3
  Rate Transition : RateTransition  OutPortSampleTime=t_sim
  Rate Transition1 : RateTransition  OutPortSampleTime=t_sim
  Rate Transition2 : RateTransition  OutPortSampleTime=t_sim
  Switch : Switch  Criteria=u2 > Threshold
  Switch1 : Switch  Criteria=u2 > Threshold
  Switch2 : Switch  Criteria=u2 > Threshold
  Noise : Outport
  wires:
  Band-Limited White Noise/1 -> Gain2/1
  Constant/1 -> Switch/2
  Constant1/1 -> Switch/3
  Gain2/1 -> Rate Transition/1
  Rate Transition/1 -> Switch/1
  Switch/1 -> Mux/1
  Mux/1 -> Noise/1
  Band-Limited White Noise1/1 -> Gain1/1
  Constant2/1 -> Switch1/2
  Constant3/1 -> Switch1/3
  Gain1/1 -> Rate Transition1/1
  Rate Transition1/1 -> Switch1/1
  Band-Limited White Noise2/1 -> Gain3/1
  Constant4/1 -> Switch2/2
  Constant5/1 -> Switch2/3
  Gain3/1 -> Rate Transition2/1
  Rate Transition2/1 -> Switch2/1
  Switch1/1 -> Mux/2
  Switch2/1 -> Mux/3

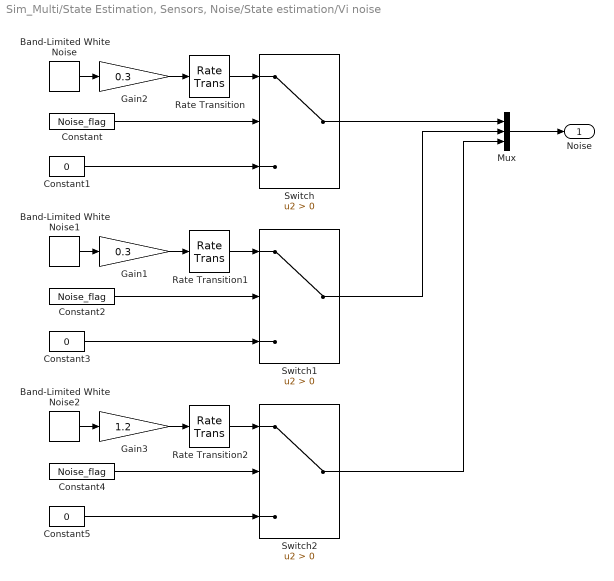
== system Sim_Multi/State Estimation, Sensors, Noise/State estimation/Vi noise ==
  Band-Limited White Noise : simulink/Sources/Band-Limited White Noise  Cov=t_sim*57.3*57.3/10000  Ts=t_sim*10  seed=[23888]
  Band-Limited White Noise1 : simulink/Sources/Band-Limited White Noise  Cov=t_sim*57.3*57.3/10000  Ts=t_sim*10  seed=[23888]
  Band-Limited White Noise2 : simulink/Sources/Band-Limited White Noise  Cov=t_sim*57.3*57.3/10000  Ts=t_sim*10  seed=[23888]
  Constant : Constant  Value=Noise_flag
  Constant1 : Constant  Value=0
  Constant2 : Constant  Value=Noise_flag
  Constant3 : Constant  Value=0
  Constant4 : Constant  Value=Noise_flag
  Constant5 : Constant  Value=0
  Gain1 : Gain  Gain=0.3
  Gain2 : Gain  Gain=0.3
  Gain3 : Gain  Gain=1.2
  Mux : Mux  Inputs=3
  Rate Transition : RateTransition  OutPortSampleTime=t_sim
  Rate Transition1 : RateTransition  OutPortSampleTime=t_sim
  Rate Transition2 : RateTransition  OutPortSampleTime=t_sim
  Switch : Switch  Criteria=u2 > Threshold
  Switch1 : Switch  Criteria=u2 > Threshold
  Switch2 : Switch  Criteria=u2 > Threshold
  Noise : Outport
  wires:
  Band-Limited White Noise/1 -> Gain2/1
  Constant/1 -> Switch/2
  Constant1/1 -> Switch/3
  Gain2/1 -> Rate Transition/1
  Rate Transition/1 -> Switch/1
  Switch/1 -> Mux/1
  Mux/1 -> Noise/1
  Band-Limited White Noise1/1 -> Gain1/1
  Constant2/1 -> Switch1/2
  Constant3/1 -> Switch1/3
  Gain1/1 -> Rate Transition1/1
  Rate Transition1/1 -> Switch1/1
  Band-Limited White Noise2/1 -> Gain3/1
  Constant4/1 -> Switch2/2
  Constant5/1 -> Switch2/3
  Gain3/1 -> Rate Transition2/1
  Rate Transition2/1 -> Switch2/1
  Switch1/1 -> Mux/2
  Switch2/1 -> Mux/3

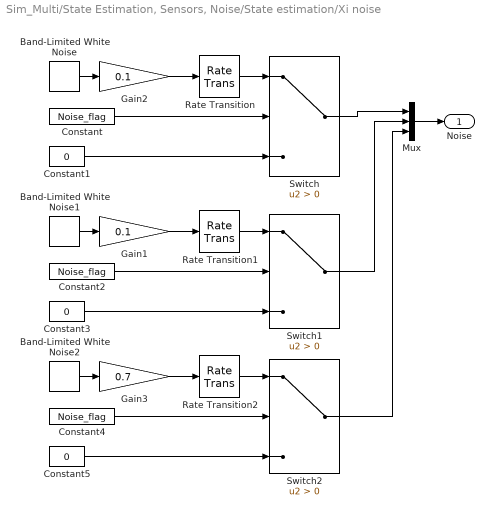
== system Sim_Multi/State Estimation, Sensors, Noise/State estimation/Xi noise ==
  Band-Limited White Noise : simulink/Sources/Band-Limited White Noise  Cov=t_sim*57.3*57.3/10000  Ts=t_sim*20  seed=[23559]
  Band-Limited White Noise1 : simulink/Sources/Band-Limited White Noise  Cov=t_sim*57.3*57.3/10000  Ts=t_sim*20  seed=[23559]
  Band-Limited White Noise2 : simulink/Sources/Band-Limited White Noise  Cov=t_sim*57.3*57.3/10000  Ts=t_sim*20  seed=[23559]
  Constant : Constant  Value=Noise_flag
  Constant1 : Constant  Value=0
  Constant2 : Constant  Value=Noise_flag
  Constant3 : Constant  Value=0
  Constant4 : Constant  Value=Noise_flag
  Constant5 : Constant  Value=0
  Gain1 : Gain  Gain=0.1
  Gain2 : Gain  Gain=0.1
  Gain3 : Gain  Gain=0.7
  Mux : Mux  Inputs=3
  Rate Transition : RateTransition  OutPortSampleTime=t_sim
  Rate Transition1 : RateTransition  OutPortSampleTime=t_sim
  Rate Transition2 : RateTransition  OutPortSampleTime=t_sim
  Switch : Switch  Criteria=u2 > Threshold
  Switch1 : Switch  Criteria=u2 > Threshold
  Switch2 : Switch  Criteria=u2 > Threshold
  Noise : Outport
  wires:
  Band-Limited White Noise/1 -> Gain2/1
  Constant/1 -> Switch/2
  Constant1/1 -> Switch/3
  Gain2/1 -> Rate Transition/1
  Mux/1 -> Noise/1
  Switch/1 -> Mux/1
  Band-Limited White Noise1/1 -> Gain1/1
  Constant2/1 -> Switch1/2
  Constant3/1 -> Switch1/3
  Gain1/1 -> Rate Transition1/1
  Band-Limited White Noise2/1 -> Gain3/1
  Constant4/1 -> Switch2/2
  Constant5/1 -> Switch2/3
  Gain3/1 -> Rate Transition2/1
  Switch1/1 -> Mux/2
  Switch2/1 -> Mux/3
  Rate Transition/1 -> Switch/1
  Rate Transition1/1 -> Switch1/1
  Rate Transition2/1 -> Switch2/1

== system Sim_Multi/True dynamic system representation of a multirotor UAV/6DOF model/Body to Inertial ==
  V_b : Inport
  DCM_ib : Inport  Port=2
  Math Function2 : Math  Operator=transpose  SaturateOnIntegerOverflow=on
  Product : Product  Multiplication=Matrix(*)
  Reshape : Reshape  OutputDimensionality=Column vector (2-D)
  Reshape1 : Reshape  OutputDimensionality=Column vector (2-D)
  V_i : Outport
  wires:
  Reshape/1 -> Product/2
  Product/1 -> Reshape1/1
  DCM_ib/1 -> Math Function2/1
  Reshape1/1 -> V_i/1
  V_b/1 -> Reshape/1
  Math Function2/1 -> Product/1  "DCM_bi"

== system Sim_Multi/True dynamic system representation of a multirotor UAV/6DOF model/Body to Inertial1 ==
  a_b : Inport
  DCM_ib : Inport  Port=2
  Math Function2 : Math  Operator=transpose  SaturateOnIntegerOverflow=on
  Product : Product  Multiplication=Matrix(*)
  Reshape : Reshape  OutputDimensionality=Column vector (2-D)
  Reshape1 : Reshape  OutputDimensionality=Column vector (2-D)
  a_i : Outport
  wires:
  Reshape/1 -> Product/2
  Product/1 -> Reshape1/1
  DCM_ib/1 -> Math Function2/1
  Reshape1/1 -> a_i/1
  a_b/1 -> Reshape/1
  Math Function2/1 -> Product/1  "DCM_bi"

== system Sim_Multi/True dynamic system representation of a multirotor UAV/6DOF model/Calculate omega_dot ==
  omega [rad/s] : Inport
  Inertia [kgm^2] : Inport  Port=2
  Moments [Nm] : Inport  Port=3
  Cross Product omega x (J * omega) : Subsystem
  Product : Product  Inputs=/*  Multiplication=Matrix(*)
  Reshape : Reshape  OutputDimensionality=Column vector (2-D)
  "Reshape " : Reshape  OutputDimensionality=Column vector (2-D)
  Subsystem : Subsystem
  Sum1 : Sum  Inputs=-+|
  omega_dot [rad/s^2] : Outport
  wires:
  Inertia [kgm^2]/1 -> Product/1, Subsystem/2(J)
  omega [rad/s]/1 -> Cross Product omega x (J * omega)/1(omega), Subsystem/1(omega)
  Subsystem/1(J * omega) -> Cross Product omega x (J * omega)/2(J * omega)
  Cross Product omega x (J * omega)/1(omega x (J * omega)) -> Reshape/1
  Product/1 -> "Reshape "/1
  "Reshape "/1 -> omega_dot [rad/s^2]/1
  Moments [Nm]/1 -> Sum1/2
  Reshape/1 -> Sum1/1
  Sum1/1 -> Product/2

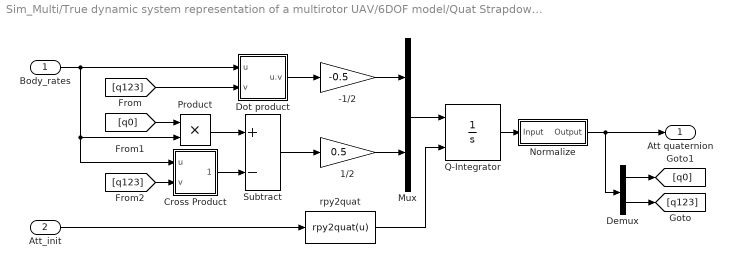
== system Sim_Multi/True dynamic system representation of a multirotor UAV/6DOF model/Quat Strapdown Eq. ==
  Body_rates : Inport
  Att_init : Inport  Port=2
  -1/2 : Gain  Gain=-0.5
  1/2 : Gain  Gain=0.5
  Cross Product : Subsystem
  Demux : Demux  Outputs=[1 3]
  Dot product : Subsystem
  Mux : Mux  Inputs=[1 3]
  Normalize : Subsystem
  Product : Product  RndMeth=Zero
  Q-Integrator : Integrator  InitialConditionSource=external  InitialCondition=[1 0 0 0]
  Subtract : Sum  Inputs=+-
  rpy2quat : MATLABFcn  MATLABFcn=rpy2quat(u)  OutputDimensions=4
  Att quaternion : Outport
  wires:
  Dot product/1(u.v) -> -1/2/1
  -1/2/1 -> Mux/1
  Body_rates/1 -> Dot product/1(u), Cross Product/1(u), Product/2
  Q-Integrator/1 -> Normalize/1(Input)
  [q123] -> Dot product/2(v)
  Product/1 -> Subtract/1
  Cross Product/1(u x v) -> Subtract/2
  [q0] -> Product/1
  [q123] -> Cross Product/2(v)
  Subtract/1 -> 1/2/1
  1/2/1 -> Mux/2
  Demux/1 -> [q0]
  Demux/2 -> [q123]
  Normalize/1(Output) -> Demux/1, Att quaternion/1
  Mux/1 -> Q-Integrator/1
  rpy2quat/1 -> Q-Integrator/2
  Att_init/1 -> rpy2quat/1

== system Sim_Multi/True dynamic system representation of a multirotor UAV/6DOF model/Quat to Euler ==
  Quaternion q : Inport
  Fcn : Fcn  Expr=2*(u(3)*u(4)+u(1)*u(2))
  Fcn1 : Fcn  Expr=2*(u(2)*u(4)-u(1)*u(3))
  Fcn2 : Fcn  Expr=2*(u(2)*u(3)+u(1)*u(4))
  Fcn3 : Fcn  Expr=u(1)*u(1)-u(2)*u(2)-u(3)*u(3)+u(4)*u(4)
  Fcn4 : Fcn  Expr=u(1)*u(1)+u(2)*u(2)-u(3)*u(3)-u(4)*u(4)
  Gain : Gain  Gain=-1
  Reshape : Reshape  OutputDimensionality=Column vector (2-D)
  Trigonometric Function : Trigonometry  Operator=asin
  Trigonometric Function1 : Trigonometry  Operator=atan2
  Trigonometric Function2 : Trigonometry  Operator=atan2
  Vector Concatenate : Concatenate  NumInputs=3
  Euler [rad] : Outport
  wires:
  Fcn1/1 -> Trigonometric Function/1
  Trigonometric Function/1 -> Gain/1
  Fcn/1 -> Trigonometric Function1/1
  Fcn3/1 -> Trigonometric Function1/2
  Fcn2/1 -> Trigonometric Function2/1
  Fcn4/1 -> Trigonometric Function2/2
  Trigonometric Function1/1 -> Vector Concatenate/1
  Gain/1 -> Vector Concatenate/2
  Trigonometric Function2/1 -> Vector Concatenate/3
  Quaternion q/1 -> Fcn4/1, Fcn2/1, Fcn/1, Fcn3/1, Fcn1/1
  Vector Concatenate/1 -> Reshape/1
  Reshape/1 -> Euler [rad]/1

== system Sim_Multi/True dynamic system representation of a multirotor UAV/6DOF model/Quat to Rotation Matrix ==
  Quaternion q : Inport
  Subsystem : Subsystem
  Subsystem1 : Subsystem
  Subsystem2 : Subsystem
  Subsystem3 : Subsystem
  Subsystem4 : Subsystem
  Subsystem5 : Subsystem
  Subsystem6 : Subsystem
  Subsystem7 : Subsystem
  Subsystem8 : Subsystem
  Subsystem9 : Subsystem
  DCM_ib : Outport
  wires:
  Quaternion q/1 -> Subsystem2/1(q), Subsystem8/1(q), Subsystem7/1(q), Subsystem6/1(q), Subsystem1/1(q), Subsystem5/1(q), Subsystem4/1(q), Subsystem3/1(q), Subsystem/1(q)
  Subsystem/1(C_11) -> Subsystem9/1(C_11)
  Subsystem3/1(C_12) -> Subsystem9/2(C_12)
  Subsystem4/1(C_13) -> Subsystem9/3(C_13)
  Subsystem5/1(C_21) -> Subsystem9/4(C_21)
  Subsystem1/1(C_22) -> Subsystem9/5(C_22)
  Subsystem2/1(C_33) -> Subsystem9/9(C_33)
  Subsystem8/1(C_32) -> Subsystem9/8(C_32)
  Subsystem7/1(C_31) -> Subsystem9/7(C_31)
  Subsystem6/1(C_23) -> Subsystem9/6(C_23)
  Subsystem9/1(DCM_ib) -> DCM_ib/1

== system Sim_Multi/True dynamic system representation of a multirotor UAV/6DOF model/omega x V_b ==
  V_b : Inport
  omega : Inport  Port=2
  Subsystem : Subsystem
  Subsystem1 : Subsystem
  Sum : Sum  Inputs=+|-
  omega x V_b : Outport
  wires:
  Sum/1 -> omega x V_b/1
  omega/1 -> Subsystem1/1(u), Subsystem/1(u)
  V_b/1 -> Subsystem/2(v), Subsystem1/2(v)
  Subsystem/1(Positive elements) -> Sum/1
  Subsystem1/1(Negative elements) -> Sum/2

== system Sim_Multi/True dynamic system representation of a multirotor UAV/Force//Moment computation/Compute aerodynamic drag of the airframe in Body axes ==
  note: Aerodynamic drag force acting on the airframe
      | The assumption is that the surface area of the airframe from different directions
      | can be described by an ellipsoid. Then the 'acting 'surface area is in the direction
      | of the airspeed vector and can be computed by scaling the airspeed vector so that
      | it points onto the surface of the ellipsoid.
  6DOF dynamics : Inport
  Dynamic parameters : Inport  Port=2
  Aerodynamic drag force : Subsystem
  Bus Selector2 : BusSelector  OutputSignals=V_b,DCM_ib
  Bus Selector3 : BusSelector  OutputSignals=Wind_i,Surface_params
  Total airspeed (Body axes) : Subsystem
  Drag force : Outport
  wires:
  Aerodynamic drag force/1(Drag force (Body axes)) -> Drag force/1
  6DOF dynamics/1 -> Bus Selector2/1
  Dynamic parameters/1 -> Bus Selector3/1
  Bus Selector3/2 -> Aerodynamic drag force/2(Surface_params)  "<Surface_params>"
  Bus Selector2/1 -> Total airspeed (Body axes)/1(V_b)  "<V_b>"
  Bus Selector2/2 -> Total airspeed (Body axes)/2(DCM_ib)  "<DCM_ib>"
  Bus Selector3/1 -> Total airspeed (Body axes)/3(Wind_i)  "<Wind_i>"
  Total airspeed (Body axes)/1(Airspeed (Body)) -> Aerodynamic drag force/1(Airspeed (Body axes))

== system Sim_Multi/True dynamic system representation of a multirotor UAV/Force//Moment computation/Compute force of gravity in Body axes ==
  note: Force of gravity acting on the airframe
  6DOF dynamics : Inport
  Dynamic parameters : Inport  Port=2
  Bus Selector : BusSelector  OutputSignals=DCM_ib
  Bus Selector1 : BusSelector  OutputSignals=mass_real
  Gravity (Inertial axes) : Constant  Value=[0;0;g]
  Product : Product  Multiplication=Matrix(*)  SaturateOnIntegerOverflow=on  InputSameDT=on  OutDataTypeStr=Inherit: Same as first input
  Product1 : Product
  Reshape : Reshape  OutputDimensionality=Column vector (2-D)
  Gravity force : Outport
  wires:
  Gravity (Inertial axes)/1 -> Product1/1
  Product1/1 -> Product/2  "Force of gravity (Inertial axes)"
  Product/1 -> Reshape/1  "Force of gravity (Body axes)"
  Reshape/1 -> Gravity force/1
  6DOF dynamics/1 -> Bus Selector/1
  Dynamic parameters/1 -> Bus Selector1/1
  Bus Selector1/1 -> Product1/2  "<mass_real>"
  Bus Selector/1 -> Product/1  "<DCM_ib>"
